simulink model "xx"  (R2023b)
settings: Solver=VariableStepAuto  StartTime=0.0  StopTime=10.0  RelTol=1e-3
settings Model: Creator=lyan  LastModifiedBy=lyan
settings ConfigComp: DVTestSuiteOptimization=Auto  DVDetectOutOfBounds=on  DVModelReferenceHarness=on  DVHarnessSource=Signal Editor  DVRebuildModelRepresentation=IfChangeIsDetected
settings ConfigsetCC: ModelAdvisorConfigurationFile=C:\MATLAB_Doc\test\xxx\MACustomChecks\myChecks\mychecks.json

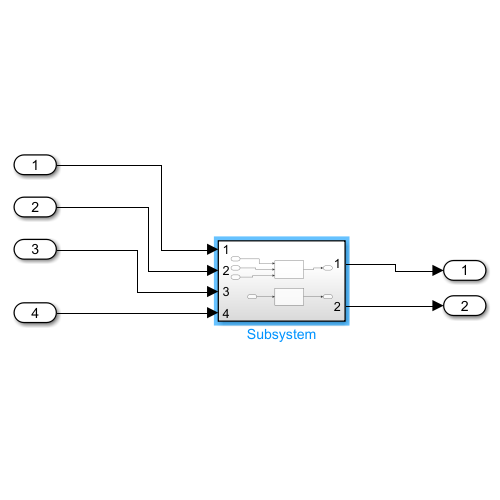
[thumbnail: Simulink's stored preview of the top-level diagram]
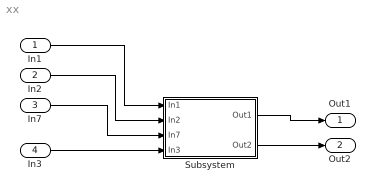
== system xx ==
  In1 : Inport
  In2 : Inport  Port=2
  In7 : Inport  Port=3
  In3 : Inport  Port=4
  Subsystem : Subsystem
  Out1 : Outport
  Out2 : Outport  Port=2
  wires:
  In7/1 -> Subsystem/3(In7)
  In2/1 -> Subsystem/2(In2)
  Subsystem/1(Out1) -> Out1/1
  Subsystem/2(Out2) -> Out2/1
  In3/1 -> Subsystem/4(In3)
  In1/1 -> Subsystem/1(In1)

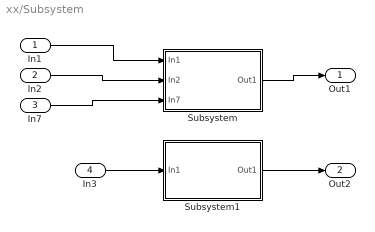
== system xx/Subsystem ==
  In1 : Inport
  In2 : Inport  Port=2
  In7 : Inport  Port=3
  In3 : Inport  Port=4
  Subsystem : Subsystem
  Subsystem1 : Subsystem
  Out1 : Outport
  Out2 : Outport  Port=2
  wires:
  In1/1 -> Subsystem/1(In1)
  Subsystem/1(Out1) -> Out1/1
  In2/1 -> Subsystem/2(In2)
  In7/1 -> Subsystem/3(In7)
  In3/1 -> Subsystem1/1(In1)
  Subsystem1/1(Out1) -> Out2/1

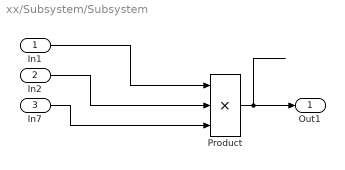
== system xx/Subsystem/Subsystem ==
  In1 : Inport
  In2 : Inport  Port=2
  In7 : Inport  Port=3
  Product : Product  Inputs=3
  Out1 : Outport
  wires:
  In1/1 -> Product/1
  In2/1 -> Product/2
  In7/1 -> Product/3
  Product/1 -> Out1/1
  ? -> ?

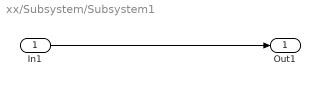
== system xx/Subsystem/Subsystem1 ==
  In1 : Inport
  Out1 : Outport
  wires:
  In1/1 -> Out1/1
